simulink subsystem "AUVPlant"  (R2024a)
settings: Solver=VariableStepAuto  StartTime=0.0  StopTime=10.0  RelTol=1e-3
undefined symbols (not defined in the file): DiscIntNeverNeededParam, dmax, dmin, dSeedX, dts, MPC, N, physics, PWM, RPM, simulation, simulink, T200, tmax, tmin, Xi
libraries: simulink x5, aerolibutil x5, embmathops x2, sharedtransform x1
settings Model: Creator=lamarre  LastModifiedBy=relat
settings SolverCC: AlgebraicLoopSolver=TrustRegion
settings DebuggingCC: UnconnectedInputMsg=warning  UnconnectedOutputMsg=warning  UnconnectedLineMsg=warning
settings ModelReferenceCC: EnableRefExpFcnMdlSchedulingChecks=on
settings RTWCC: GPUComputeCapability=3.5  DLArmComputeVersion=19.05

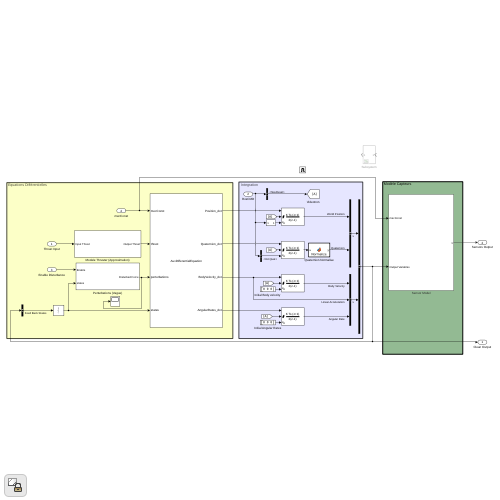
[thumbnail: Simulink's stored preview of the top-level diagram]
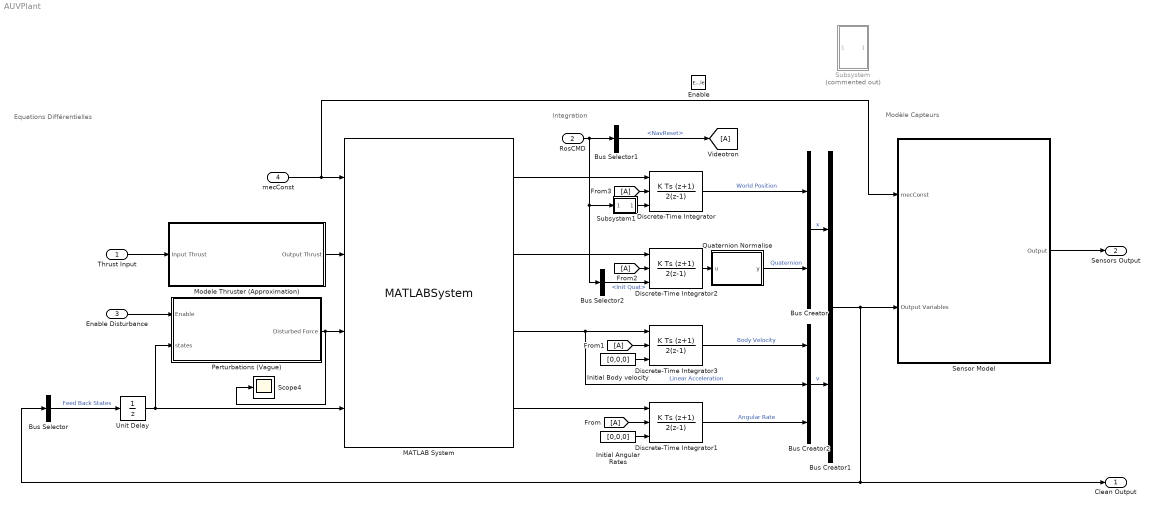
== system AUVPlant ==
  note: Modèle Capteurs
  note: Equations Différentielles
  note: Integration
  Thrust Input : Inport
  RosCMD : Inport  Port=2
  Enable Disturbance : Inport  Port=3
  mecConst : Inport  Port=4
  Enable : EnablePort
  Bus Creator : BusCreator  Inputs=2
  Bus Creator1 : BusCreator  Inputs=2
  Bus Creator2 : BusCreator  Inputs=3
  Bus Selector : BusSelector  OutputSignals=x.World Position,x.Quaternion,v.Body Velocity,v.Angular Rate  OutputAsBus=on
  Bus Selector1 : BusSelector  OutputSignals=NavReset
  Bus Selector2 : BusSelector  OutputSignals=Init Quat
  Discrete-Time Integrator{,1..3} (4 alike) : DiscreteIntegrator  IntegratorMethod=Integration: Trapezoidal  ExternalReset=rising  InitialConditionSource=external  SampleTime=simulink.sampletime  ICPrevOutput=DiscIntNeverNeededParam  ICPrevScaledInput=DiscIntNeverNeededParam
  From{,1..3} (4 alike) : From
  Initial Angular Rates : Constant  Value=[0,0,0]
  "Initial Body velocity " : Constant  Value=[0,0,0]
  MATLAB System : MATLABSystem  System=AuvDifferentialEquation  simulation=simulation  MPC=MPC  useDynamicsConst=on  SimulateUsing=Code generation
      mask Type: AuvDifferentialEquation
      mask Display:
      | disp('AuvDifferentialEquation');
      | port_label('input',1,'mecConst');
      | port_label('input',2,'thrust');
      | port_label('input',3,'perturbations');
      | port_label('input',4,'states');
      | port_label('output',1,'Position_dot');
      | port_label('output',2,'Quaternion_dot');
      | port_label('output',3,'BodyVelocity_dot');
      | port_label('output',4,'AngularRates_dot');
  Modele Thruster (Approximation) : Subsystem
  Perturbations (Vague) : Subsystem
  Quaternion Normalise : MATLAB Function  TreatAsAtomicUnit=on
  Scope4 : Scope
  Sensor Model : Subsystem
  Subsystem : Subsystem  Commented=on
  Subsystem1 : Subsystem
  Unit Delay : UnitDelay  InitialCondition=MPC.Xi  SampleTime=simulink.sampletime  HasFrameUpgradeWarning=on
  Videotron : Goto
  Clean Output : Outport
  Sensors Output : Outport  Port=2
  wires:
  "Initial Body velocity "/1 -> Discrete-Time Integrator3/3
  MATLAB System/2 -> Discrete-Time Integrator2/1
  Discrete-Time Integrator/1 -> Bus Creator/1  "World Position"
  Discrete-Time Integrator3/1 -> Bus Creator2/1  "Body Velocity"
  MATLAB System/1 -> Discrete-Time Integrator/1
  Initial Angular Rates/1 -> Discrete-Time Integrator1/3
  MATLAB System/4 -> Discrete-Time Integrator1/1
  Discrete-Time Integrator1/1 -> Bus Creator2/3  "Angular Rate"
  Bus Selector2/1 -> Discrete-Time Integrator2/3  "<Init Quat>"
  MATLAB System/3 -> Bus Creator2/2, Discrete-Time Integrator3/1  "Linear Acceleration"
  From/1 -> Discrete-Time Integrator1/2
  From1/1 -> Discrete-Time Integrator3/2
  From2/1 -> Discrete-Time Integrator2/2
  From3/1 -> Discrete-Time Integrator/2
  Sensor Model/1(Output) -> Sensors Output/1
  Discrete-Time Integrator2/1 -> Quaternion Normalise/1(u)
  Quaternion Normalise/1(y) -> Bus Creator/2  "Quaternion"
  Perturbations (Vague)/1(Disturbed Force) -> MATLAB System/3, Scope4/1
  Bus Creator/1 -> Bus Creator1/1  "x"
  Bus Creator2/1 -> Bus Creator1/2  "v"
  Enable Disturbance/1 -> Perturbations (Vague)/1(Enable)
  Thrust Input/1 -> Modele Thruster (Approximation)/1(Input Thrust)
  Modele Thruster (Approximation)/1(Output Thrust) -> MATLAB System/2
  Bus Creator1/1 -> Sensor Model/2(Output Variables), Bus Selector/1, Clean Output/1
  Bus Selector/1 -> Unit Delay/1  "Feed Back States"
  Unit Delay/1 -> MATLAB System/4, Perturbations (Vague)/2(states)
  RosCMD/1 -> Bus Selector1/1, Subsystem1/1(In1), Bus Selector2/1
  Bus Selector1/1 -> Videotron/1  "<NavReset>"
  Subsystem1/1(Out1) -> Discrete-Time Integrator/3
  mecConst/1 -> MATLAB System/1, Sensor Model/1(mecConst)

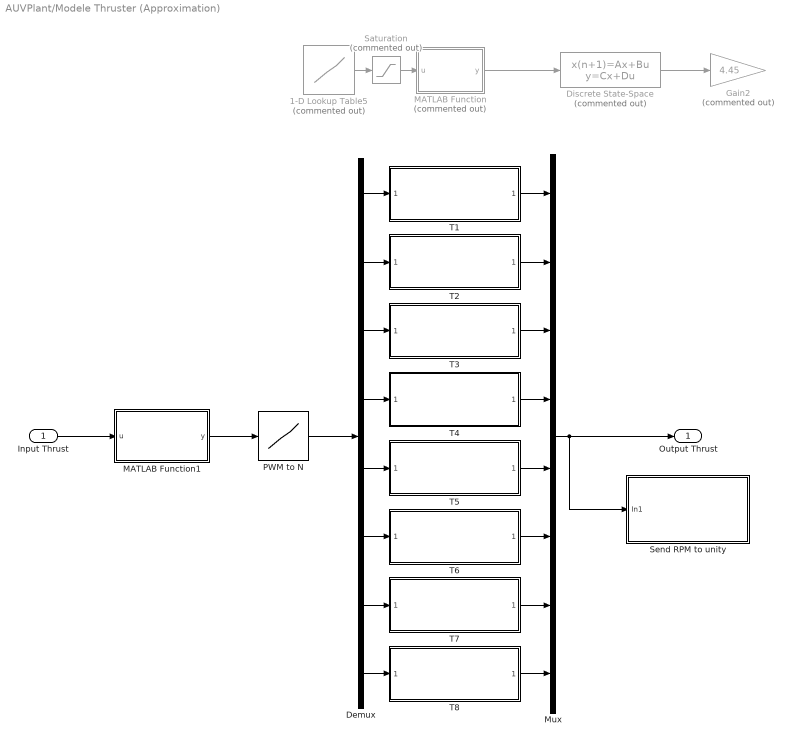
== system AUVPlant/Modele Thruster (Approximation) ==
  Input Thrust : Inport
  " PWM to N" : Lookup_n-D  NumberOfTableDimensions=1  BreakpointsForDimension1=PWM  BreakpointsForDimension1DataTypeStr=uint16  BeginIndexSearchUsingPreviousIndexResult=on  Table=N  TableDataTypeStr=double  InterpMethod=Nearest  ExtrapMethod=Clip  InternalRulePriority=Speed  OutDataTypeStr=double  RndMeth=Simplest
  1-D Lookup Table5 : Lookup_n-D  Commented=on  NumberOfTableDimensions=1  BreakpointsForDimension1=N  Table=PWM  InterpMethod=Nearest  InternalRulePriority=Speed  RndMeth=Simplest
  Demux : Demux  Outputs=8
  Discrete State-Space : DiscreteStateSpace  Commented=on  A=T200.A  B=T200.B  C=T200.C  D=T200.D  SampleTime=T200.Ts
  Gain2 : Gain  Commented=on  Gain=4.45
  MATLAB Function : MATLAB Function  Commented=on  TreatAsAtomicUnit=on
  MATLAB Function1 : MATLAB Function  TreatAsAtomicUnit=on
  Mux : Mux  Inputs=8
  Saturation : Saturate  Commented=on  UpperLimit=tmax  LowerLimit=tmin  LinearizeAsGain=off  ZeroCross=off
  Send RPM to unity : Subsystem
  T{1..8} (8 alike) : Subsystem  ReferencedSubsystem=ThrusterModel
  Output Thrust : Outport
  wires:
  MATLAB Function1/1(y) -> " PWM to N"/1
  Input Thrust/1 -> MATLAB Function1/1(u)
  " PWM to N"/1 -> Demux/1
  Saturation/1 -> MATLAB Function/1(u)
  1-D Lookup Table5/1 -> Saturation/1
  Discrete State-Space/1 -> Gain2/1
  MATLAB Function/1(y) -> Discrete State-Space/1
  Demux/1 -> T1/1
  Demux/2 -> T2/1
  Demux/3 -> T3/1
  Demux/4 -> T4/1
  Demux/5 -> T5/1
  Demux/6 -> T6/1
  Demux/8 -> T8/1
  Demux/7 -> T7/1
  T1/1 -> Mux/1
  T2/1 -> Mux/2
  T3/1 -> Mux/3
  T4/1 -> Mux/4
  T5/1 -> Mux/5
  T6/1 -> Mux/6
  T7/1 -> Mux/7
  T8/1 -> Mux/8
  Mux/1 -> Output Thrust/1, Send RPM to unity/1(In1)

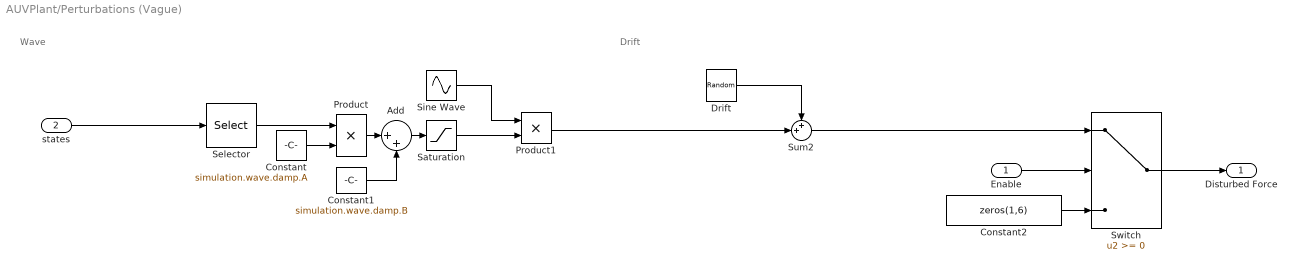
== system AUVPlant/Perturbations (Vague) ==
  note: Drift
  note: Wave
  Enable : Inport
  states : Inport  Port=2
  " Drift" : UniformRandomNumber  Minimum=dmin  Maximum=dmax  Seed=dSeedX  SampleTime=dts
  Add : Sum  Inputs=|++
  Constant : Constant  Value=simulation.wave.damp.A
  Constant1 : Constant  Value=simulation.wave.damp.B
  Constant2 : Constant  Value=zeros(1,6)
  Product : Product
  Product1 : Product
  Saturation : Saturate  UpperLimit=simulation.wave.damp.min  LowerLimit=simulation.wave.damp.max
  Selector : Selector  InputPortWidth=13  IndexOptions=Index vector (dialog)  Indices=[ 3]  OutputSizes=1
  Sine Wave : Sin  SineType=Sample based  Amplitude=simulation.wave.amplitudes  Samples=waveDiscreteFrequency  SampleTime=simulink.sampletime  Offset=waveDiscretePhase
  Sum2 : Sum  Inputs=++|
  Switch : Switch  SaturateOnIntegerOverflow=off  InputSameDT=off
  Disturbed Force : Outport
  wires:
  " Drift"/1 -> Sum2/1
  Sine Wave/1 -> Product1/1
  Enable/1 -> Switch/2
  Switch/1 -> Disturbed Force/1
  Constant2/1 -> Switch/3
  Saturation/1 -> Product1/2
  Add/1 -> Saturation/1
  Product1/1 -> Sum2/2
  Constant1/1 -> Add/2
  Product/1 -> Add/1
  Selector/1 -> Product/1
  Constant/1 -> Product/2
  states/1 -> Selector/1
  Sum2/1 -> Switch/1

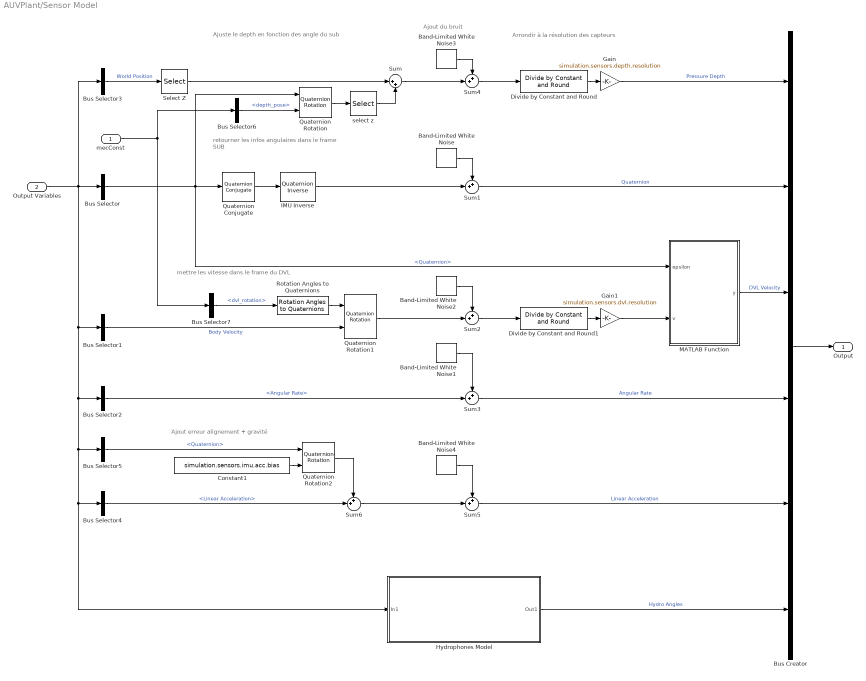
== system AUVPlant/Sensor Model ==
  note: retourner les infos
      | angulaires dans
      | le frame SUB
  note: mettre les vitesse dans le frame du DVL
  note: Ajout du bruit
  note: Ajuste le depth en fonction des angle du sub
  note: Arrondir à la résolution des capteurs
  note: Ajout erreur alignement + gravité
  mecConst : Inport
  Output Variables : Inport  Port=2
  Band-Limited White Noise : simulink/Sources/Band-Limited White Noise  Cov=[simulation.sensors.noise.power]  Ts=simulation.sensors.noise.sampletime  seed=[23341]
  Band-Limited White Noise1 : simulink/Sources/Band-Limited White Noise  Cov=[simulation.sensors.imu.gyro.noisePower]  Ts=simulation.sensors.noise.sampletime  seed=[23341]
  Band-Limited White Noise2 : simulink/Sources/Band-Limited White Noise  Cov=[simulation.sensors.dvl.noise.power]  Ts=simulation.sensors.noise.sampletime  seed=[23341]
  Band-Limited White Noise3 : simulink/Sources/Band-Limited White Noise  Cov=[simulation.sensors.noise.power]  Ts=simulation.sensors.noise.sampletime  seed=[23341]
  Band-Limited White Noise4 : simulink/Sources/Band-Limited White Noise  Cov=[simulation.sensors.imu.acc.noisePower]  Ts=simulation.sensors.noise.sampletime  seed=[23341]
  Bus Creator : BusCreator  Inputs=6
  Bus Selector : BusSelector  OutputSignals=x.Quaternion
  Bus Selector1 : BusSelector  OutputSignals=v.Body Velocity  OutputAsBus=on
  Bus Selector2 : BusSelector  OutputSignals=v.Angular Rate
  Bus Selector3 : BusSelector  OutputSignals=x.World Position  OutputAsBus=on
  Bus Selector4 : BusSelector  OutputSignals=v.Linear Acceleration
  Bus Selector5 : BusSelector  OutputSignals=x.Quaternion
  Bus Selector6 : BusSelector  OutputSignals=depth_pose
  Bus Selector7 : BusSelector  OutputSignals=dvl_rotation
  Constant1 : Constant  Value=simulation.sensors.imu.acc.bias
  Divide by Constant and Round : embmathops/Divide by Constant and Round  Denominator=simulation.sensors.depth.resolution  RoundingMethod=Nearest  SimulateUsing=Code generation
  Divide by Constant and Round1 : embmathops/Divide by Constant and Round  Denominator=simulation.sensors.dvl.resolution  RoundingMethod=Nearest  SimulateUsing=Code generation
  Gain : Gain  Gain=simulation.sensors.depth.resolution
  Gain1 : Gain  Gain=simulation.sensors.dvl.resolution
  Hydrophones Model : Subsystem
  IMU Inverse : aerolibutil/Quaternion Inverse
  MATLAB Function : MATLAB Function  TreatAsAtomicUnit=on
  Quaternion Conjugate : aerolibutil/Quaternion Conjugate
  Quaternion Rotation : aerolibutil/Quaternion Rotation
  Quaternion Rotation1 : aerolibutil/Quaternion Rotation
  Quaternion Rotation2 : aerolibutil/Quaternion Rotation
  Rotation Angles to Quaternions : sharedtransform/Rotation Angles to Quaternions  rotationOrder=XYZ  aMode=aMode
  Select Z : Selector  InputPortWidth=3  IndexOptions=Index vector (dialog)  Indices=[3]  OutputSizes=1
  Sum : Sum  Inputs=|++
  Sum{1..6} (6 alike) : Sum  Inputs=++|
  select z : Selector  InputPortWidth=3  IndexOptions=Index vector (dialog)  Indices=[3]  OutputSizes=1
  Output : Outport
  wires:
  mecConst/1 -> Bus Selector6/1, Bus Selector7/1
  Hydrophones Model/1(Out1) -> Bus Creator/6  "Hydro Angles"
  Output Variables/1 -> Bus Selector3/1, Bus Selector1/1, Bus Selector2/1, Bus Selector4/1, Hydrophones Model/1(In1), Bus Selector5/1, Bus Selector/1
  Band-Limited White Noise1/1 -> Sum3/1
  Band-Limited White Noise/1 -> Sum1/1
  Bus Selector4/1 -> Sum6/2  "<Linear Acceleration>"
  Sum6/1 -> Sum5/2
  Quaternion Rotation2/1 -> Sum6/1
  Bus Selector5/1 -> Quaternion Rotation2/1  "<Quaternion>"
  Constant1/1 -> Quaternion Rotation2/2
  Sum5/1 -> Bus Creator/5  "Linear Acceleration"
  Band-Limited White Noise4/1 -> Sum5/1
  Divide by Constant and Round1/1 -> Gain1/1
  Gain1/1 -> MATLAB Function/2(v)
  Sum4/1 -> Divide by Constant and Round/1
  Divide by Constant and Round/1 -> Gain/1
  Band-Limited White Noise3/1 -> Sum4/1
  Sum/1 -> Sum4/2
  MATLAB Function/1(y) -> Bus Creator/3  "DVL Velocity"
  Sum2/1 -> Divide by Constant and Round1/1
  Band-Limited White Noise2/1 -> Sum2/1
  Quaternion Rotation1/1 -> Sum2/2
  Gain/1 -> Bus Creator/1  "Pressure Depth"
  select z/1 -> Sum/2
  Quaternion Rotation/1 -> select z/1
  Bus Selector6/1 -> Quaternion Rotation/2  "<depth_pose>"
  Select Z/1 -> Sum/1
  Bus Selector3/1 -> Select Z/1  "World Position"
  Quaternion Conjugate/1 -> IMU Inverse/1
  Bus Selector/1 -> Quaternion Conjugate/1, MATLAB Function/1(epsilon), Quaternion Rotation/1  "<Quaternion>"
  IMU Inverse/1 -> Sum1/2
  Rotation Angles to Quaternions/1 -> Quaternion Rotation1/1
  Bus Selector1/1 -> Quaternion Rotation1/2  "Body Velocity"
  Bus Selector7/1 -> Rotation Angles to Quaternions/1  "<dvl_rotation>"
  Sum3/1 -> Bus Creator/4  "Angular Rate"
  Sum1/1 -> Bus Creator/2  "Quaternion"
  Bus Selector2/1 -> Sum3/2  "<Angular Rate>"
  Bus Creator/1 -> Output/1

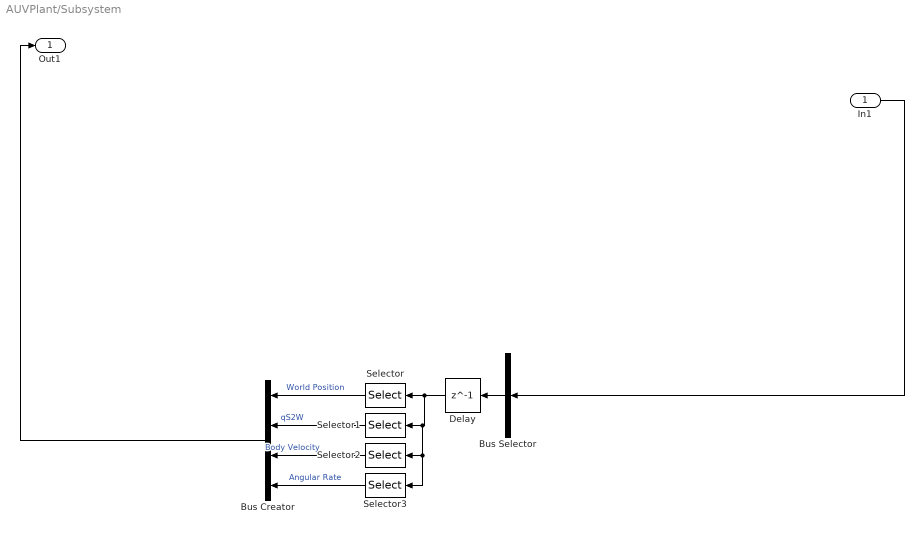
== system AUVPlant/Subsystem ==
  In1 : Inport
  Bus Creator : BusCreator  Inputs=4
  Bus Selector : BusSelector  OutputSignals=signal1.World Position,signal1.Quaternion,signal2.Body Velocity,signal2.Angular Rate  OutputAsBus=on
  Delay : Delay  DelayLength=1  InitialCondition=Xi
  Selector : Selector  InputPortWidth=13  IndexOptions=Index vector (dialog)  Indices=[1:3]  OutputSizes=1
  Selector1 : Selector  InputPortWidth=13  IndexOptions=Index vector (dialog)  Indices=[4:7]  OutputSizes=1
  Selector2 : Selector  InputPortWidth=13  IndexOptions=Index vector (dialog)  Indices=[8:10]  OutputSizes=1
  Selector3 : Selector  InputPortWidth=13  IndexOptions=Index vector (dialog)  Indices=[11:13]  OutputSizes=1
  Out1 : Outport
  wires:
  Selector3/1 -> Bus Creator/4  "Angular Rate"
  Selector2/1 -> Bus Creator/3  "Body Velocity"
  Bus Selector/1 -> Delay/1
  In1/1 -> Bus Selector/1
  Selector1/1 -> Bus Creator/2  "qS2W"
  Delay/1 -> Selector/1, Selector1/1, Selector2/1, Selector3/1
  Bus Creator/1 -> Out1/1
  Selector/1 -> Bus Creator/1  "World Position"

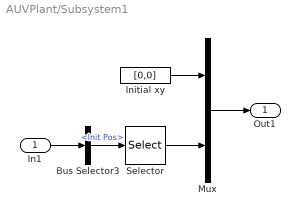
== system AUVPlant/Subsystem1 ==
  In1 : Inport
  Bus Selector3 : BusSelector  OutputSignals=Init Pos
  Initial xy : Constant  Value=[0,0]
  Mux : Mux  Inputs=2
  Selector : Selector  InputPortWidth=3  IndexOptions=Index vector (dialog)  Indices=[3]  OutputSizes=1
  Out1 : Outport
  wires:
  Selector/1 -> Mux/2
  In1/1 -> Bus Selector3/1
  Mux/1 -> Out1/1
  Initial xy/1 -> Mux/1
  Bus Selector3/1 -> Selector/1  "<Init Pos>"

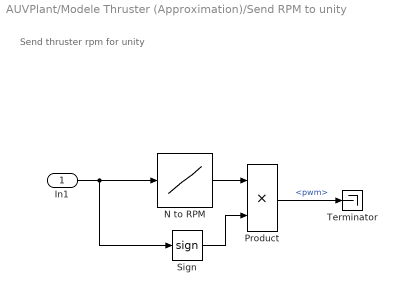
== system AUVPlant/Modele Thruster (Approximation)/Send RPM to unity ==
  note: Send thruster rpm for unity
  In1 : Inport
  N to RPM : Lookup_n-D  NumberOfTableDimensions=1  BreakpointsForDimension1=N  BreakpointsForDimension1DataTypeStr=double  BeginIndexSearchUsingPreviousIndexResult=on  Table=RPM  TableDataTypeStr=double  InterpMethod=Nearest  ExtrapMethod=Clip  InternalRulePriority=Speed  OutDataTypeStr=int16  RndMeth=Simplest
  Product : Product  OutDataTypeStr=int16
  Sign : Signum
  Terminator : Terminator
  wires:
  Product/1 -> Terminator/1  "<pwm>"
  In1/1 -> N to RPM/1, Sign/1
  N to RPM/1 -> Product/1
  Sign/1 -> Product/2

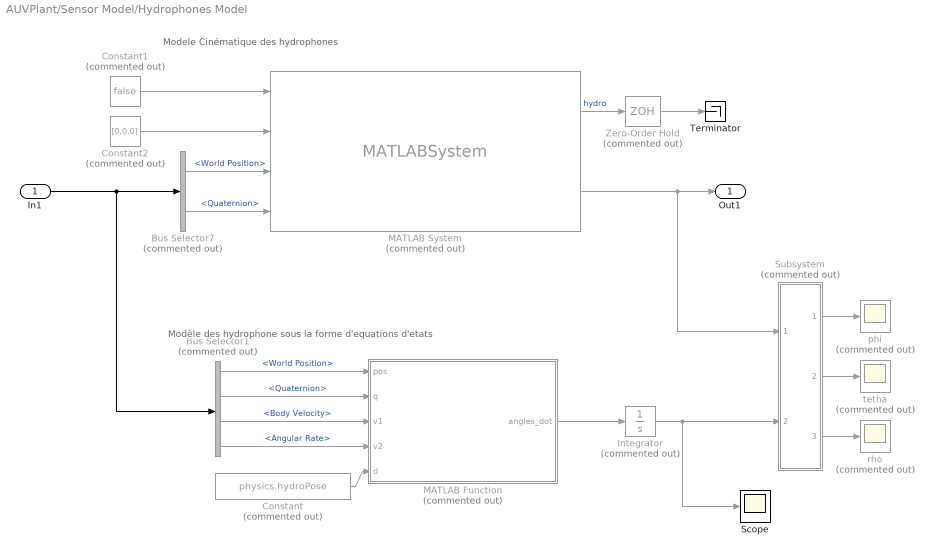
== system AUVPlant/Sensor Model/Hydrophones Model ==
  note: Modele Cinématique des hydrophones
  note: Modèle des hydrophone sous la forme d'equations d'etats
  In1 : Inport
  Bus Selector1 : BusSelector  Commented=on  OutputSignals=x.World Position,x.Quaternion,v.Body Velocity,v.Angular Rate
  Bus Selector7 : BusSelector  Commented=on  OutputSignals=x.World Position,x.Quaternion
  Constant : Constant  Commented=on  Value=physics.hydroPose
  Constant1 : Constant  Commented=on  Value=false
  Constant2 : Constant  Commented=on  Value=[0,0,0]
  Integrator : Integrator  Commented=on  InitialCondition=[1,0,9].'
  MATLAB Function : MATLAB Function  Commented=on  TreatAsAtomicUnit=on
  MATLAB System : MATLABSystem  Commented=on  System=HydroModel  Physics=physics  simulation=simulation  pingerStartPosition=[10 0 5]  SimulateUsing=Code generation
      mask Type: HydroModel
      mask Display:
      | disp('HydroModel');
      | port_label('input',1,'isNewPosition');
      | port_label('input',2,'pingerPosition');
      | port_label('input',3,'worldPosition');
      | port_label('input',4,'quaternion');
      | port_label('output',1,'pingerPosition');
      | port_label('output',2,'HydroMesurements');
  Scope : Scope
  Subsystem : Subsystem  Commented=on
  Terminator : Terminator
  Zero-Order Hold : ZeroOrderHold  Commented=on
  phi : Scope  Commented=on
  rho : Scope  Commented=on
  tetha : Scope  Commented=on
  Out1 : Outport
  wires:
  Bus Selector7/2 -> MATLAB System/4  "<Quaternion>"
  Subsystem/3(Out3) -> rho/1
  Subsystem/2(Out2) -> tetha/1
  Subsystem/1(Out1) -> phi/1
  Integrator/1 -> Scope/1, Subsystem/2(In2)
  MATLAB Function/1(angles_dot) -> Integrator/1
  Constant/1 -> MATLAB Function/5(d)
  Bus Selector1/4 -> MATLAB Function/4(v2)  "<Angular Rate>"
  Bus Selector1/3 -> MATLAB Function/3(v1)  "<Body Velocity>"
  Bus Selector1/2 -> MATLAB Function/2(q)  "<Quaternion>"
  Bus Selector1/1 -> MATLAB Function/1(pos)  "<World Position>"
  MATLAB System/1 -> Zero-Order Hold/1  "hydro"
  Constant1/1 -> MATLAB System/1
  Zero-Order Hold/1 -> Terminator/1
  In1/1 -> Bus Selector7/1, Bus Selector1/1
  MATLAB System/2 -> Out1/1, Subsystem/1(In1)
  Bus Selector7/1 -> MATLAB System/3  "<World Position>"
  Constant2/1 -> MATLAB System/2

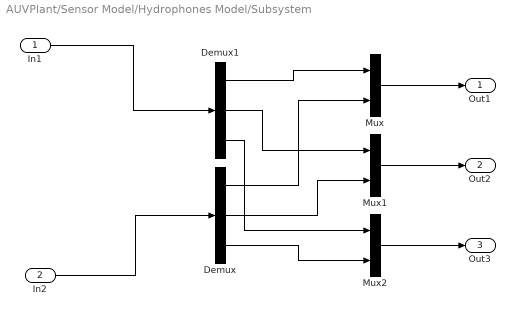
== system AUVPlant/Sensor Model/Hydrophones Model/Subsystem ==
  In1 : Inport
  In2 : Inport  Port=2
  Demux : Demux  Outputs=3
  Demux1 : Demux  Outputs=3
  Mux : Mux  Inputs=2
  Mux1 : Mux  Inputs=2
  Mux2 : Mux  Inputs=2
  Out1 : Outport
  Out2 : Outport  Port=2
  Out3 : Outport  Port=3
  wires:
  Demux1/3 -> Mux2/1
  Demux/2 -> Mux1/2
  Demux1/2 -> Mux1/1
  In2/1 -> Demux/1
  Mux/1 -> Out1/1
  Demux/3 -> Mux2/2
  In1/1 -> Demux1/1
  Demux/1 -> Mux/2
  Demux1/1 -> Mux/1
  Mux2/1 -> Out3/1
  Mux1/1 -> Out2/1

== matlab function AUVPlant/Modele Thruster (Approximation)/MATLAB Function1 ==
  data: u input; y output
function y = wrapPWM(u)
 for i=1: size(u,1)
     if u(i)<1100 || u(i)>1900
         u(i)=1500;
     end
 end
y = u;

== matlab function AUVPlant/Modele Thruster (Approximation)/MATLAB Function ==
  data: u input; y output
function y = fcn(u)
pwm=u-1500;
if pwm>=0 
    y=pwm;
else
   y=pwm*0.77969348659;
end

== matlab function AUVPlant/Quaternion Normalise ==
  data: u input size=4; y output size=4
function y = Normalize(u)
%Normailse le quaternions pour éviter la distortions crée par l'erreur de
% de l'intégration.
d=norm(u);
y = u/d;

== matlab function AUVPlant/Sensor Model/MATLAB Function ==
  data: epsilon input; y output; v input
function y = DvlLost(epsilon,v)
% This fonction simulate a ping failure if the pitch or roll angle is
% to important

e =abs(quat2eul(epsilon.','ZYX'));

if(e(2)>0.349066 || e(3)>0.349066) % If roll pitch exeed 20deg
    
    v = 32.7675*ones(3,1);
    
end

y = v;

== matlab function AUVPlant/Sensor Model/Hydrophones Model/MATLAB Function ==
  settings: updateMethod=DISCRETE
  data: pos input; angles_dot output; q input; v1 input; v2 input; d input
function angles_dot = hydro_dot(pos,q, v1, v2, d)


  angles_dot = hydroAnglesDot(pos,q.', [v1 ; v2].', d, [10, 0, 5].');
